simulink model "k1visprotoIP"  (Simulink 8.5)
settings: Solver=ode45  StartTime=0.0  StopTime=10.0  RelTol=1e-3
libraries: cdsFiltCtrl x82, cdsFilt x45, cdsMuxMatrix x18, cdsEpicsOut x7, cdsEpicsBinIn x2, cdsAdcx0 x1, dac x1, simulink x1, cdsParameters x1
(part 5 of 14)

== system k1visprotoIP/PROTO/F0/TEST ==
  Ground1 : Ground
  Ground2 : Ground
  Ground3 : Ground
  L : cdsFilt/Subsystem  Tag=cdsFilt  Description=|
      | Purpose:                                                                                                                                                                                                                                  
      | Standard CDS IIR filter module.                                                                                                                                                                                                           
      |                                                                                                                                                                                                                                           
      | Operation:                                                                                                                                                                                                                                
      | Consists of 10 second order section IIR filters, plus a ramped gain stage. In FE code, also provides pre-defined test points and excitation channel inputs. The filter coefficients are defined in the LIGO system using the 'foton' tool.
      |                                                                                                                                                                                                                                           
      | Usage:                                                                                                                                                                                                                                    
      | Name the part with the desired filter module name.
      settings: AttributesFormatString=%<Tag>
  T : cdsFilt/Subsystem  Tag=cdsFilt  Description=|
      | Purpose:                                                                                                                                                                                                                                  
      | Standard CDS IIR filter module.                                                                                                                                                                                                           
      |                                                                                                                                                                                                                                           
      | Operation:                                                                                                                                                                                                                                
      | Consists of 10 second order section IIR filters, plus a ramped gain stage. In FE code, also provides pre-defined test points and excitation channel inputs. The filter coefficients are defined in the LIGO system using the 'foton' tool.
      |                                                                                                                                                                                                                                           
      | Usage:                                                                                                                                                                                                                                    
      | Name the part with the desired filter module name.
      settings: AttributesFormatString=%<Tag>
  Y : cdsFilt/Subsystem  Tag=cdsFilt  Description=|
      | Purpose:                                                                                                                                                                                                                                  
      | Standard CDS IIR filter module.                                                                                                                                                                                                           
      |                                                                                                                                                                                                                                           
      | Operation:                                                                                                                                                                                                                                
      | Consists of 10 second order section IIR filters, plus a ramped gain stage. In FE code, also provides pre-defined test points and excitation channel inputs. The filter coefficients are defined in the LIGO system using the 'foton' tool.
      |                                                                                                                                                                                                                                           
      | Usage:                                                                                                                                                                                                                                    
      | Name the part with the desired filter module name.
      settings: AttributesFormatString=%<Tag>
  L_Out : Outport
  T_Out : Outport  Port=2
  Y_Out : Outport  Port=3
  wires:
  Ground3/1 -> Y/1
  Ground2/1 -> T/1
  Ground1/1 -> L/1
  L/1 -> L_Out/1
  T/1 -> T_Out/1
  Y/1 -> Y_Out/1

== system k1visprotoIP/PROTO/GAS/ADD ==
  LOCAL_F0_IN : Inport
  LOCAL_F1_IN : Inport  Port=2
  LOCAL_F2_IN : Inport  Port=3
  TEST_F0_IN : Inport  Port=4
  TEST_F1_IN : Inport  Port=5
  TEST_F2_IN : Inport  Port=6
  F0_MON : cdsEpicsOut/Subsystem  Tag=cdsEpicsOutput  Description=|
      | Purpose:                                          
      | Output a FE signal to an EPICS channel.           
      |                                                   
      | Operation:                                        
      | Takes input value and passes it to EPICS record.  
      |                                                   
      | Usage:                                            
      | Name the part with the desired EPICS rrecord name.
      settings: AttributesFormatString=%<Tag>
  F1_MON : cdsEpicsOut/Subsystem  Tag=cdsEpicsOutput  Description=|
      | Purpose:                                          
      | Output a FE signal to an EPICS channel.           
      |                                                   
      | Operation:                                        
      | Takes input value and passes it to EPICS record.  
      |                                                   
      | Usage:                                            
      | Name the part with the desired EPICS rrecord name.
      settings: AttributesFormatString=%<Tag>
  F2_MON : cdsEpicsOut/Subsystem  Tag=cdsEpicsOutput  Description=|
      | Purpose:                                          
      | Output a FE signal to an EPICS channel.           
      |                                                   
      | Operation:                                        
      | Takes input value and passes it to EPICS record.  
      |                                                   
      | Usage:                                            
      | Name the part with the desired EPICS rrecord name.
      settings: AttributesFormatString=%<Tag>
  Sum1 : Sum
  Sum2 : Sum
  Sum3 : Sum
  F0_OUT : Outport
  F1_OUT : Outport  Port=2
  F2_OUT : Outport  Port=3
  wires:
  TEST_F2_IN/1 -> Sum3/2
  TEST_F1_IN/1 -> Sum2/2
  TEST_F0_IN/1 -> Sum1/2
  Sum2/1 -> F1_MON/1
  Sum3/1 -> F2_MON/1
  LOCAL_F1_IN/1 -> Sum2/1
  LOCAL_F2_IN/1 -> Sum3/1
  Sum1/1 -> F0_MON/1
  LOCAL_F0_IN/1 -> Sum1/1
  F0_MON/1 -> F0_OUT/1
  F1_MON/1 -> F1_OUT/1
  F2_MON/1 -> F2_OUT/1

== system k1visprotoIP/PROTO/GAS/COILMASTER ==
  F0_IN : Inport
  F1_IN : Inport  Port=2
  F2_IN : Inport  Port=3
  SW_IN : Inport  Port=4
  Choice1 : Switch  Criteria=u2 > Threshold
  Choice2 : Switch  Criteria=u2 > Threshold
  Choice3 : Switch  Criteria=u2 > Threshold
  Ground1 : Ground
  Ground2 : Ground
  Ground3 : Ground
  F0_Out : Outport
  F1_Out : Outport  Port=2
  F2_Out : Outport  Port=3
  wires:
  Choice3/1 -> F2_Out/1
  Choice2/1 -> F1_Out/1
  Choice1/1 -> F0_Out/1
  SW_IN/1 -> Choice1/2, Choice3/2, Choice2/2
  F2_IN/1 -> Choice3/1
  Ground3/1 -> Choice3/3
  Ground2/1 -> Choice2/3
  F1_IN/1 -> Choice2/1
  Ground1/1 -> Choice1/3
  F0_IN/1 -> Choice1/1

== system k1visprotoIP/PROTO/GAS/COILOUTF ==
  F0_IN : Inport
  F1_IN : Inport  Port=2
  F2_IN : Inport  Port=3
  F0 : cdsFiltCtrl/IIR FM with control  Tag=cdsFiltCtrl  Description=|
      | cdsFiltCntrl is the standard IIR filter module (exactly the same as cdsFilt) but with added control data output 'Ctrl'. Filter module digital signal output appears on the first output, which is called 'Val'. 'Ctrl' output has a bit pattern encoding the state of filter's on/off switches (FM1 through FM10). The bit values are:
      |                                                                                                                                                                                                                                                                                                                                       
      | module 	hex	dec                                                                                                                                                                                                                                                                                                                       
      | -----------------------                                                                                                                                                                                                                                                                                                               
      | FM1	0x20                    32                                                                                                                                                                                                                                                                                                        
      | FM2	0x80                     128                                                                                                                                                                                                                                                                                                      
      | FM3	0x200                   512                                                                                                                                                                                                                                                                                                       
      | FM4	0x800                   2048                                                                                                                                                                                                                                                                                                      
      | FM5	0x2000                 8192                                                                                                                                                                                                                                                                                                       
      | FM6	0x8000                 32768                                                                                                                                                                                                                                                                                                      
      | FM7	0x20000                131072                                                                                                                                                                                                                                                                                                     
      | FM8	0x80000                 524288                                                                                                                                                                                                                                                                                                    
      | FM9	0x200000               2097152                                                                                                                                                                                                                                                                                                    
      | FM10	0x800000               8388608                                                                                                                                                                                                                                                                                                   
      |                                                                                                                                                                                                                                                                                                                                       
      | This bit data can be used to drive some other switches or it can be output using a binary I/O module.
      settings: AttributesFormatString=%<Tag>
  F1 : cdsFiltCtrl/IIR FM with control  Tag=cdsFiltCtrl  Description=|
      | cdsFiltCntrl is the standard IIR filter module (exactly the same as cdsFilt) but with added control data output 'Ctrl'. Filter module digital signal output appears on the first output, which is called 'Val'. 'Ctrl' output has a bit pattern encoding the state of filter's on/off switches (FM1 through FM10). The bit values are:
      |                                                                                                                                                                                                                                                                                                                                       
      | module 	hex	dec                                                                                                                                                                                                                                                                                                                       
      | -----------------------                                                                                                                                                                                                                                                                                                               
      | FM1	0x20                    32                                                                                                                                                                                                                                                                                                        
      | FM2	0x80                     128                                                                                                                                                                                                                                                                                                      
      | FM3	0x200                   512                                                                                                                                                                                                                                                                                                       
      | FM4	0x800                   2048                                                                                                                                                                                                                                                                                                      
      | FM5	0x2000                 8192                                                                                                                                                                                                                                                                                                       
      | FM6	0x8000                 32768                                                                                                                                                                                                                                                                                                      
      | FM7	0x20000                131072                                                                                                                                                                                                                                                                                                     
      | FM8	0x80000                 524288                                                                                                                                                                                                                                                                                                    
      | FM9	0x200000               2097152                                                                                                                                                                                                                                                                                                    
      | FM10	0x800000               8388608                                                                                                                                                                                                                                                                                                   
      |                                                                                                                                                                                                                                                                                                                                       
      | This bit data can be used to drive some other switches or it can be output using a binary I/O module.
      settings: AttributesFormatString=%<Tag>
  F2 : cdsFiltCtrl/IIR FM with control  Tag=cdsFiltCtrl  Description=|
      | cdsFiltCntrl is the standard IIR filter module (exactly the same as cdsFilt) but with added control data output 'Ctrl'. Filter module digital signal output appears on the first output, which is called 'Val'. 'Ctrl' output has a bit pattern encoding the state of filter's on/off switches (FM1 through FM10). The bit values are:
      |                                                                                                                                                                                                                                                                                                                                       
      | module 	hex	dec                                                                                                                                                                                                                                                                                                                       
      | -----------------------                                                                                                                                                                                                                                                                                                               
      | FM1	0x20                    32                                                                                                                                                                                                                                                                                                        
      | FM2	0x80                     128                                                                                                                                                                                                                                                                                                      
      | FM3	0x200                   512                                                                                                                                                                                                                                                                                                       
      | FM4	0x800                   2048                                                                                                                                                                                                                                                                                                      
      | FM5	0x2000                 8192                                                                                                                                                                                                                                                                                                       
      | FM6	0x8000                 32768                                                                                                                                                                                                                                                                                                      
      | FM7	0x20000                131072                                                                                                                                                                                                                                                                                                     
      | FM8	0x80000                 524288                                                                                                                                                                                                                                                                                                    
      | FM9	0x200000               2097152                                                                                                                                                                                                                                                                                                    
      | FM10	0x800000               8388608                                                                                                                                                                                                                                                                                                   
      |                                                                                                                                                                                                                                                                                                                                       
      | This bit data can be used to drive some other switches or it can be output using a binary I/O module.
      settings: AttributesFormatString=%<Tag>
  Ground1 : Ground
  Ground2 : Ground
  Ground3 : Ground
  Terminator1 : Terminator
  Terminator2 : Terminator
  Terminator3 : Terminator
  F0_Out : Outport
  F1_Out : Outport  Port=2
  F2_Out : Outport  Port=3
  wires:
  F0/2 -> Terminator1/1
  Ground1/1 -> F0/2
  F0_IN/1 -> F0/1
  F1/2 -> Terminator2/1
  Ground2/1 -> F1/2
  F1_IN/1 -> F1/1
  F2/2 -> Terminator3/1
  Ground3/1 -> F2/2
  F2_IN/1 -> F2/1
  F0/1 -> F0_Out/1
  F1/1 -> F1_Out/1
  F2/1 -> F2_Out/1

== system k1visprotoIP/PROTO/GAS/LVDTINF ==
  F0_IN : Inport
  F1_IN : Inport  Port=2
  F2_IN : Inport  Port=3
  F0 : cdsFiltCtrl/IIR FM with control  Tag=cdsFiltCtrl  Description=|
      | cdsFiltCntrl is the standard IIR filter module (exactly the same as cdsFilt) but with added control data output 'Ctrl'. Filter module digital signal output appears on the first output, which is called 'Val'. 'Ctrl' output has a bit pattern encoding the state of filter's on/off switches (FM1 through FM10). The bit values are:
      |                                                                                                                                                                                                                                                                                                                                       
      | module 	hex	dec                                                                                                                                                                                                                                                                                                                       
      | -----------------------                                                                                                                                                                                                                                                                                                               
      | FM1	0x20                    32                                                                                                                                                                                                                                                                                                        
      | FM2	0x80                     128                                                                                                                                                                                                                                                                                                      
      | FM3	0x200                   512                                                                                                                                                                                                                                                                                                       
      | FM4	0x800                   2048                                                                                                                                                                                                                                                                                                      
      | FM5	0x2000                 8192                                                                                                                                                                                                                                                                                                       
      | FM6	0x8000                 32768                                                                                                                                                                                                                                                                                                      
      | FM7	0x20000                131072                                                                                                                                                                                                                                                                                                     
      | FM8	0x80000                 524288                                                                                                                                                                                                                                                                                                    
      | FM9	0x200000               2097152                                                                                                                                                                                                                                                                                                    
      | FM10	0x800000               8388608                                                                                                                                                                                                                                                                                                   
      |                                                                                                                                                                                                                                                                                                                                       
      | This bit data can be used to drive some other switches or it can be output using a binary I/O module.
      settings: AttributesFormatString=%<Tag>
  F1 : cdsFiltCtrl/IIR FM with control  Tag=cdsFiltCtrl  Description=|
      | cdsFiltCntrl is the standard IIR filter module (exactly the same as cdsFilt) but with added control data output 'Ctrl'. Filter module digital signal output appears on the first output, which is called 'Val'. 'Ctrl' output has a bit pattern encoding the state of filter's on/off switches (FM1 through FM10). The bit values are:
      |                                                                                                                                                                                                                                                                                                                                       
      | module 	hex	dec                                                                                                                                                                                                                                                                                                                       
      | -----------------------                                                                                                                                                                                                                                                                                                               
      | FM1	0x20                    32                                                                                                                                                                                                                                                                                                        
      | FM2	0x80                     128                                                                                                                                                                                                                                                                                                      
      | FM3	0x200                   512                                                                                                                                                                                                                                                                                                       
      | FM4	0x800                   2048                                                                                                                                                                                                                                                                                                      
      | FM5	0x2000                 8192                                                                                                                                                                                                                                                                                                       
      | FM6	0x8000                 32768                                                                                                                                                                                                                                                                                                      
      | FM7	0x20000                131072                                                                                                                                                                                                                                                                                                     
      | FM8	0x80000                 524288                                                                                                                                                                                                                                                                                                    
      | FM9	0x200000               2097152                                                                                                                                                                                                                                                                                                    
      | FM10	0x800000               8388608                                                                                                                                                                                                                                                                                                   
      |                                                                                                                                                                                                                                                                                                                                       
      | This bit data can be used to drive some other switches or it can be output using a binary I/O module.
      settings: AttributesFormatString=%<Tag>
  F2 : cdsFiltCtrl/IIR FM with control  Tag=cdsFiltCtrl  Description=|
      | cdsFiltCntrl is the standard IIR filter module (exactly the same as cdsFilt) but with added control data output 'Ctrl'. Filter module digital signal output appears on the first output, which is called 'Val'. 'Ctrl' output has a bit pattern encoding the state of filter's on/off switches (FM1 through FM10). The bit values are:
      |                                                                                                                                                                                                                                                                                                                                       
      | module 	hex	dec                                                                                                                                                                                                                                                                                                                       
      | -----------------------                                                                                                                                                                                                                                                                                                               
      | FM1	0x20                    32                                                                                                                                                                                                                                                                                                        
      | FM2	0x80                     128                                                                                                                                                                                                                                                                                                      
      | FM3	0x200                   512                                                                                                                                                                                                                                                                                                       
      | FM4	0x800                   2048                                                                                                                                                                                                                                                                                                      
      | FM5	0x2000                 8192                                                                                                                                                                                                                                                                                                       
      | FM6	0x8000                 32768                                                                                                                                                                                                                                                                                                      
      | FM7	0x20000                131072                                                                                                                                                                                                                                                                                                     
      | FM8	0x80000                 524288                                                                                                                                                                                                                                                                                                    
      | FM9	0x200000               2097152                                                                                                                                                                                                                                                                                                    
      | FM10	0x800000               8388608                                                                                                                                                                                                                                                                                                   
      |                                                                                                                                                                                                                                                                                                                                       
      | This bit data can be used to drive some other switches or it can be output using a binary I/O module.
      settings: AttributesFormatString=%<Tag>
  Ground1 : Ground
  Ground2 : Ground
  Ground3 : Ground
  Terminator1 : Terminator
  Terminator2 : Terminator
  Terminator3 : Terminator
  F0_OUT : Outport
  F1_OUT : Outport  Port=2
  F2_OUT : Outport  Port=3
  wires:
  F2/2 -> Terminator3/1
  F2/1 -> F2_OUT/1
  Ground3/1 -> F2/2
  F2_IN/1 -> F2/1
  F1/2 -> Terminator2/1
  F1/1 -> F1_OUT/1
  Ground2/1 -> F1/2
  F1_IN/1 -> F1/1
  F0/2 -> Terminator1/1
  F0/1 -> F0_OUT/1
  Ground1/1 -> F0/2
  F0_IN/1 -> F0/1
